simulink model "feedback_model"  (R2022a)
settings: Solver=VariableStepAuto  StartTime=0.0  StopTime=0.2  RelTol=1e-3
settings Model: Creator=novik  LastModifiedBy=novik

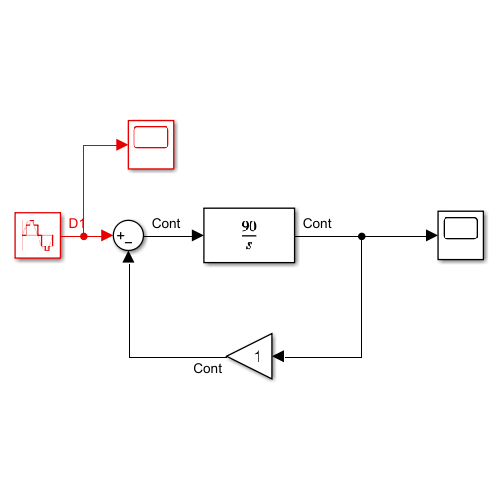
[thumbnail: Simulink's stored preview of the top-level diagram]
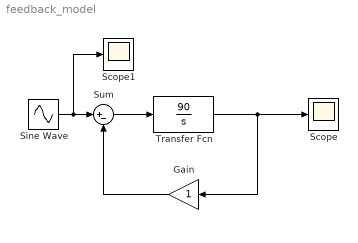
== system feedback_model ==
  Gain : Gain
  Scope : Scope
  Scope1 : Scope
  Sine Wave : Sin  Amplitude=100  Frequency=1800  SampleTime=0.000001
  Sum : Sum  Inputs=|+-
  Transfer Fcn : TransferFcn  Numerator=[90]  Denominator=[1 0]
  wires:
  Transfer Fcn/1 -> Gain/1, Scope/1
  Sine Wave/1 -> Scope1/1, Sum/1
  Sum/1 -> Transfer Fcn/1
  Gain/1 -> Sum/2
